simulink model "v1"  (R2025b)
settings: Solver=VariableStepAuto  StartTime=0.0  StopTime=100  RelTol=1e-3
libraries: uavutilslib x1
settings Model: Creator=hamza  LastModifiedBy=hamza

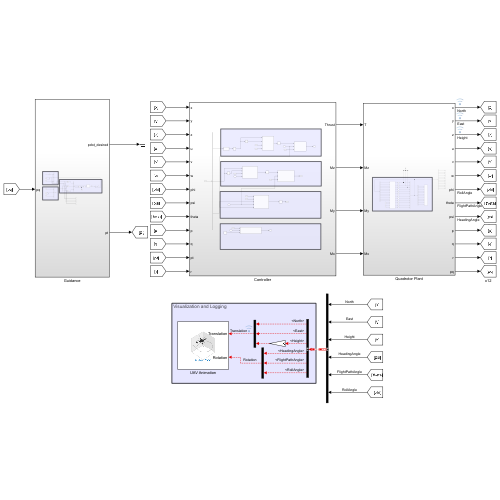
[thumbnail: Simulink's stored preview of the top-level diagram]
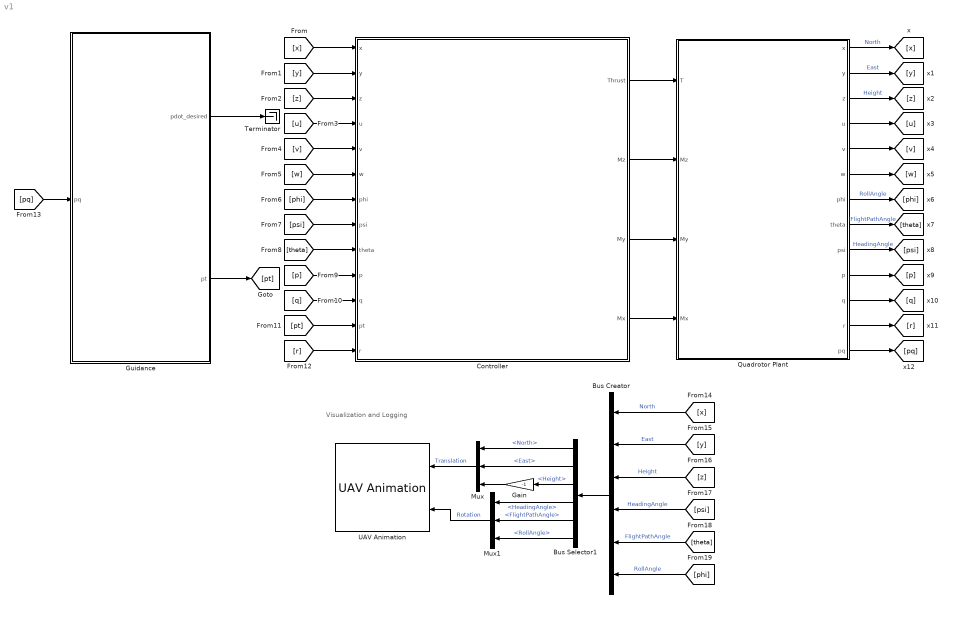
== system v1 ==
  note: Visualization and Logging
  Bus Creator : BusCreator  Inputs=6
  Bus Selector1 : BusSelector  OutputSignals=North,East,Height,HeadingAngle,FlightPathAngle,RollAngle
  Controller : Subsystem
  Gain : Gain  Gain=-1
  Guidance : Subsystem
  Mux : Mux  Inputs=3
  Mux1 : Mux  Inputs=3
  Quadrotor Plant : Subsystem
  Terminator : Terminator
  UAV Animation : uavutilslib/UAV Animation  NumUAV=1  DynamicUAVConfig=off  UAVType=Multirotor  UAVSize=5  UAVColor=[1 0 0]  UAVTrajectoryAlpha=1  InertialZDirection=Down  RotationFormat=Euler ZYX  DrawMarkers=off  SampleTime=0.1
  wires:
  Guidance/1(pdot_desired) -> Terminator/1
  Controller/1(Thrust) -> Quadrotor Plant/1(T)
  Controller/2(Mz) -> Quadrotor Plant/2(Mz)
  Controller/3(My) -> Quadrotor Plant/3(My)
  Controller/4(Mx) -> Quadrotor Plant/4(Mx)
  Mux1/1 -> UAV Animation/2  "Rotation"
  Gain/1 -> Mux/3
  Bus Selector1/1 -> Mux/1  "<North>"
  Bus Selector1/6 -> Mux1/3  "<RollAngle>"
  Mux/1 -> UAV Animation/1  "Translation"
  Bus Selector1/3 -> Gain/1  "<Height>"
  Bus Selector1/2 -> Mux/2  "<East>"
  Bus Selector1/4 -> Mux1/1  "<HeadingAngle>"
  Bus Selector1/5 -> Mux1/2  "<FlightPathAngle>"
  Bus Creator/1 -> Bus Selector1/1
  [x] -> Controller/1(x)
  [y] -> Controller/2(y)
  [z] -> Controller/3(z)
  [u] -> Controller/4(u)
  [v] -> Controller/5(v)
  [w] -> Controller/6(w)
  [phi] -> Controller/7(phi)
  [psi] -> Controller/8(psi)
  [theta] -> Controller/9(theta)
  [p] -> Controller/10(p)
  [q] -> Controller/11(q)
  [pt] -> Controller/12(pt)
  [r] -> Controller/13(r)
  Quadrotor Plant/1(x) -> [x]  "North"
  Quadrotor Plant/2(y) -> [y]  "East"
  Quadrotor Plant/3(z) -> [z]  "Height"
  Quadrotor Plant/4(u) -> [u]
  Quadrotor Plant/5(v) -> [v]
  Quadrotor Plant/6(w) -> [w]
  Quadrotor Plant/7(phi) -> [phi]  "RollAngle"
  Quadrotor Plant/8(theta) -> [theta]  "FlightPathAngle"
  Quadrotor Plant/9(psi) -> [psi]  "HeadingAngle"
  Quadrotor Plant/10(p) -> [p]
  Quadrotor Plant/11(q) -> [q]
  Quadrotor Plant/12(r) -> [r]
  Quadrotor Plant/13(pq) -> [pq]
  Guidance/2(pt) -> [pt]
  [pq] -> Guidance/1(pq)
  [phi] -> Bus Creator/6  "RollAngle"
  [theta] -> Bus Creator/5  "FlightPathAngle"
  [psi] -> Bus Creator/4  "HeadingAngle"
  [z] -> Bus Creator/3  "Height"
  [y] -> Bus Creator/2  "East"
  [x] -> Bus Creator/1  "North"

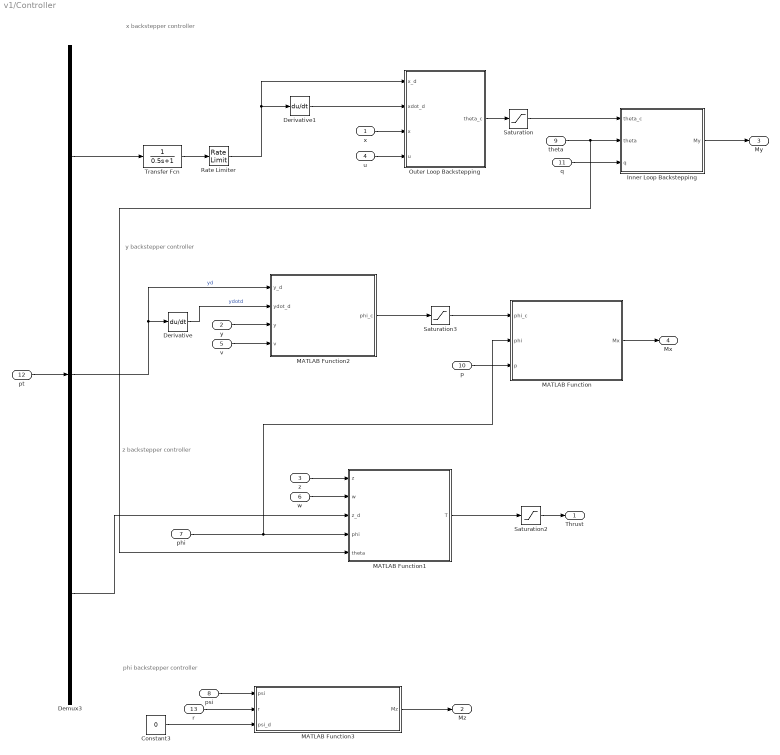
== system v1/Controller ==
  note: phi backstepper controller
  note: z backstepper controller
  note: y backstepper controller
  note: x backstepper controller
  x : Inport
  y : Inport  Port=2
  z : Inport  Port=3
  u : Inport  Port=4
  v : Inport  Port=5
  w : Inport  Port=6
  phi : Inport  Port=7
  psi : Inport  Port=8
  theta : Inport  Port=9
  p : Inport  Port=10
  q : Inport  Port=11
  pt : Inport  Port=12
  r : Inport  Port=13
  Constant3 : Constant  Value=0
  Demux3 : Demux  Outputs=3
  Derivative : Derivative
  Derivative1 : Derivative
  Inner Loop Backstepping : MATLAB Function  TreatAsAtomicUnit=on
  MATLAB Function : MATLAB Function  TreatAsAtomicUnit=on
  MATLAB Function1 : MATLAB Function  TreatAsAtomicUnit=on
  MATLAB Function2 : MATLAB Function  TreatAsAtomicUnit=on
  MATLAB Function3 : MATLAB Function  TreatAsAtomicUnit=on
  Outer Loop Backstepping : MATLAB Function  TreatAsAtomicUnit=on
  Rate Limiter : RateLimiter  RisingSlewLimit=0.5  FallingSlewLimit=-0.5  SampleTimeMode=inherited
  Saturation : Saturate  UpperLimit=0.1  LowerLimit=-0.1
  Saturation2 : Saturate  UpperLimit=22  LowerLimit=0
  Saturation3 : Saturate  UpperLimit=0.1  LowerLimit=-0.1
  Transfer Fcn : TransferFcn  Denominator=[0.5 1]
  Thrust : Outport
  Mz : Outport  Port=2
  My : Outport  Port=3
  Mx : Outport  Port=4
  wires:
  z/1 -> MATLAB Function1/1(z)
  x/1 -> Outer Loop Backstepping/3(x)
  Saturation/1 -> Inner Loop Backstepping/1(theta_c)
  Inner Loop Backstepping/1(My) -> My/1
  Constant3/1 -> MATLAB Function3/3(psi_d)
  Saturation3/1 -> MATLAB Function/1(phi_c)
  phi/1 -> MATLAB Function/2(phi), MATLAB Function1/4(phi)
  Demux3/1 -> Transfer Fcn/1
  Demux3/2 -> MATLAB Function2/1(y_d), Derivative/1  "yd"
  Demux3/3 -> MATLAB Function1/3(z_d)
  MATLAB Function2/1(phi_c) -> Saturation3/1
  r/1 -> MATLAB Function3/2(r)
  MATLAB Function3/1(Mz) -> Mz/1
  y/1 -> MATLAB Function2/3(y)
  Outer Loop Backstepping/1(theta_c) -> Saturation/1
  MATLAB Function1/1(T) -> Saturation2/1
  v/1 -> MATLAB Function2/4(v)
  w/1 -> MATLAB Function1/2(w)
  Derivative/1 -> MATLAB Function2/2(ydot_d)  "ydotd"
  pt/1 -> Demux3/1
  psi/1 -> MATLAB Function3/1(psi)
  u/1 -> Outer Loop Backstepping/4(u)
  theta/1 -> MATLAB Function1/5(theta), Inner Loop Backstepping/2(theta)
  MATLAB Function/1(Mx) -> Mx/1
  q/1 -> Inner Loop Backstepping/3(q)
  p/1 -> MATLAB Function/3(p)
  Saturation2/1 -> Thrust/1
  Derivative1/1 -> Outer Loop Backstepping/2(xdot_d)
  Transfer Fcn/1 -> Rate Limiter/1
  Rate Limiter/1 -> Outer Loop Backstepping/1(x_d), Derivative1/1

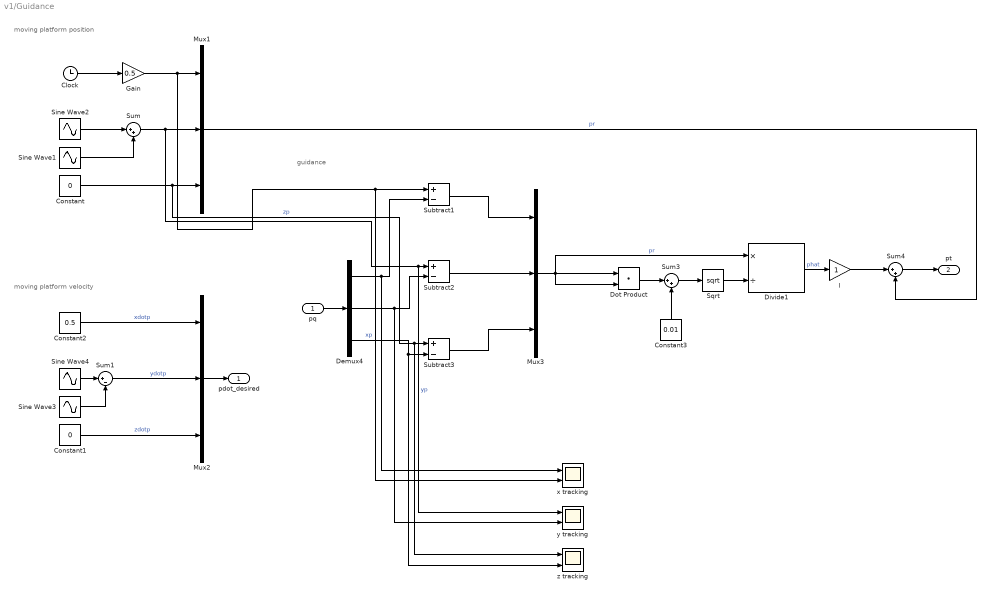
== system v1/Guidance ==
  note: guidance
  note: moving platform position
  note: moving platform velocity
  pq : Inport
  Clock : Clock
  Constant : Constant  Value=0
  Constant1 : Constant  Value=0
  Constant2 : Constant  Value=0.5
  Constant3 : Constant  Value=0.01
  Demux4 : Demux  Outputs=3
  Divide1 : Product  Inputs=*/
  Dot Product : DotProduct  OutDataTypeStr=Inherit: Inherit via internal rule
  Gain : Gain  Gain=0.5
  Mux1 : Mux  Inputs=3
  Mux2 : Mux  Inputs=3
  Mux3 : Mux  Inputs=3
  Sine Wave1 : Sin  Amplitude=2  Frequency=0.2  SampleTime=0
  Sine Wave2 : Sin  Amplitude=2  Frequency=0.2  Phase=pi/2  SampleTime=0
  Sine Wave3 : Sin  Amplitude=0.4  Frequency=0.2  SampleTime=0
  Sine Wave4 : Sin  Amplitude=0.4  Frequency=0.2  Phase=pi/2  SampleTime=0
  Sqrt : Sqrt
  Subtract1 : Sum  Inputs=+-
  Subtract2 : Sum  Inputs=+-
  Subtract3 : Sum  Inputs=+-
  Sum : Sum  Inputs=|++
  Sum1 : Sum  Inputs=|+-
  Sum3 : Sum  Inputs=|++
  Sum4 : Sum  Inputs=|++
  l : Gain
  x tracking : Scope  NumInputPorts=2
      settings: ActiveDisplayYMinimum=-1  ActiveDisplayYMaximum=1  DataLoggingVariableName=ScopeData5
  y tracking : Scope  NumInputPorts=2
      settings: ActiveDisplayYMinimum=-6.2686091559816877  ActiveDisplayYMaximum=6.2529287715888877  DataLoggingVariableName=ScopeData6
  z tracking : Scope  NumInputPorts=2
      settings: ActiveDisplayYMinimum=-1  ActiveDisplayYMaximum=1  DataLoggingVariableName=ScopeData7
  pdot_desired : Outport
  pt : Outport  Port=2
  wires:
  Sine Wave3/1 -> Sum1/2
  Mux1/1 -> Sum4/2  "pr"
  Sine Wave1/1 -> Sum/2
  Constant2/1 -> Mux2/1  "xdotp"
  Constant/1 -> z tracking/1, Subtract3/1, Mux1/3  "zp"
  Sum1/1 -> Mux2/2  "ydotp"
  pq/1 -> Demux4/1
  Sine Wave4/1 -> Sum1/1
  Constant1/1 -> Mux2/3  "zdotp"
  Clock/1 -> Gain/1
  Gain/1 -> x tracking/2, Subtract1/1, Mux1/1  "xp"
  Sum/1 -> y tracking/1, Subtract2/1, Mux1/2  "yp"
  Mux2/1 -> pdot_desired/1
  Sine Wave2/1 -> Sum/1
  Demux4/1 -> x tracking/1, Subtract1/2
  Demux4/2 -> y tracking/2, Subtract2/2
  Demux4/3 -> z tracking/2, Subtract3/2
  Subtract2/1 -> Mux3/2
  Subtract3/1 -> Mux3/3
  Subtract1/1 -> Mux3/1
  Mux3/1 -> Dot Product/1, Divide1/1, Dot Product/2  "pr"
  Dot Product/1 -> Sum3/1
  Constant3/1 -> Sum3/2
  Sum3/1 -> Sqrt/1
  Sqrt/1 -> Divide1/2
  Divide1/1 -> l/1  "phat"
  l/1 -> Sum4/1
  Sum4/1 -> pt/1

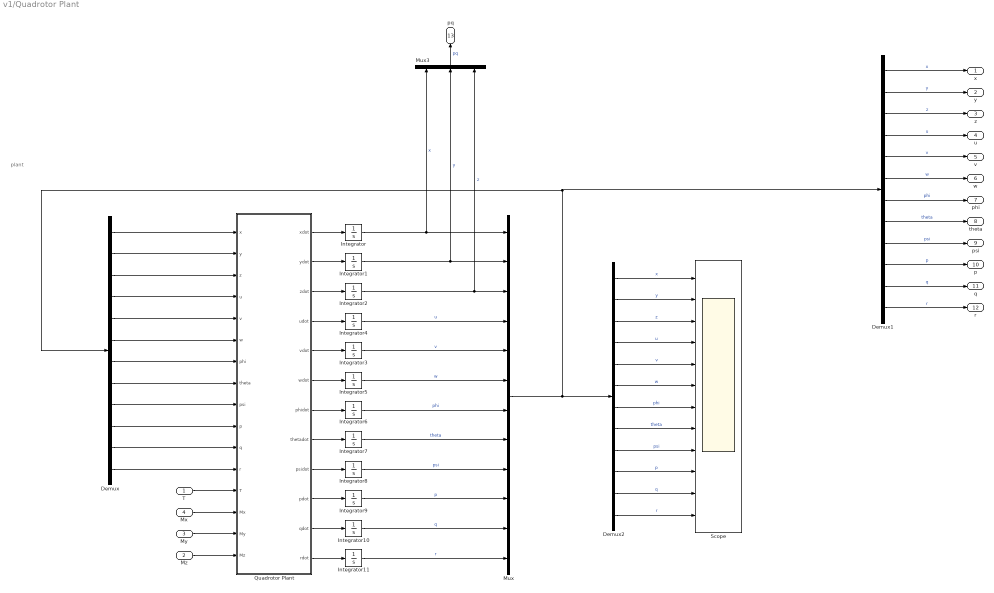
== system v1/Quadrotor Plant ==
  note: plant
  T : Inport
  Mz : Inport  Port=2
  My : Inport  Port=3
  Mx : Inport  Port=4
  Demux : Demux  Outputs=12
  Demux1 : Demux  Outputs=12
  Demux2 : Demux  Outputs=12
  Integrator{,1..11} (12 alike) : Integrator
  Mux : Mux  Inputs=12
  Mux3 : Mux  Inputs=3
  Quadrotor Plant : MATLAB Function  TreatAsAtomicUnit=on
  Scope : Scope  NumInputPorts=12
      settings: ActiveDisplayString=12  ActiveDisplayYMinimum=-1  ActiveDisplayYMaximum=1
  x : Outport
  y : Outport  Port=2
  z : Outport  Port=3
  u : Outport  Port=4
  v : Outport  Port=5
  w : Outport  Port=6
  phi : Outport  Port=7
  theta : Outport  Port=8
  psi : Outport  Port=9
  p : Outport  Port=10
  q : Outport  Port=11
  r : Outport  Port=12
  pq : Outport  Port=13
  wires:
  Demux2/8 -> Scope/8  "theta"
  Demux2/11 -> Scope/11  "q"
  Integrator3/1 -> Mux/5  "v"
  Demux2/5 -> Scope/5  "v"
  Demux/1 -> Quadrotor Plant/1(x)
  Integrator/1 -> Mux/1, Mux3/1  "x"
  Mux/1 -> Demux2/1, Demux1/1, Demux/1
  Integrator2/1 -> Mux3/3, Mux/3  "z"
  Demux/8 -> Quadrotor Plant/8(theta)
  Quadrotor Plant/4(udot) -> Integrator4/1
  Demux/9 -> Quadrotor Plant/9(psi)
  Integrator1/1 -> Mux/2, Mux3/2  "y"
  Demux/6 -> Quadrotor Plant/6(w)
  Quadrotor Plant/12(rdot) -> Integrator11/1
  Quadrotor Plant/5(vdot) -> Integrator3/1
  Demux2/9 -> Scope/9  "psi"
  Integrator5/1 -> Mux/6  "w"
  Quadrotor Plant/9(psidot) -> Integrator8/1
  Demux/4 -> Quadrotor Plant/4(u)
  Demux/12 -> Quadrotor Plant/12(r)
  Quadrotor Plant/2(ydot) -> Integrator1/1
  Mz/1 -> Quadrotor Plant/16(Mz)
  Quadrotor Plant/1(xdot) -> Integrator/1
  Integrator4/1 -> Mux/4  "u"
  Demux2/10 -> Scope/10  "p"
  Demux2/3 -> Scope/3  "z"
  Demux/11 -> Quadrotor Plant/11(q)
  Demux2/6 -> Scope/6  "w"
  Demux/2 -> Quadrotor Plant/2(y)
  Demux2/4 -> Scope/4  "u"
  Integrator8/1 -> Mux/9  "psi"
  Integrator10/1 -> Mux/11  "q"
  Demux/10 -> Quadrotor Plant/10(p)
  Demux2/1 -> Scope/1  "x"
  Quadrotor Plant/10(pdot) -> Integrator9/1
  Mx/1 -> Quadrotor Plant/14(Mx)
  Demux2/2 -> Scope/2  "y"
  Quadrotor Plant/7(phidot) -> Integrator6/1
  Integrator7/1 -> Mux/8  "theta"
  Mux3/1 -> pq/1  "pq"
  Integrator11/1 -> Mux/12  "r"
  Demux2/12 -> Scope/12  "r"
  Demux/5 -> Quadrotor Plant/5(v)
  T/1 -> Quadrotor Plant/13(T)
  Integrator9/1 -> Mux/10  "p"
  Demux/7 -> Quadrotor Plant/7(phi)
  Quadrotor Plant/8(thetadot) -> Integrator7/1
  Quadrotor Plant/3(zdot) -> Integrator2/1
  Demux2/7 -> Scope/7  "phi"
  Demux/3 -> Quadrotor Plant/3(z)
  Quadrotor Plant/6(wdot) -> Integrator5/1
  Quadrotor Plant/11(qdot) -> Integrator10/1
  My/1 -> Quadrotor Plant/15(My)
  Integrator6/1 -> Mux/7  "phi"
  Demux1/1 -> x/1  "x"
  Demux1/2 -> y/1  "y"
  Demux1/3 -> z/1  "z"
  Demux1/4 -> u/1  "u"
  Demux1/5 -> v/1  "v"
  Demux1/6 -> w/1  "w"
  Demux1/7 -> phi/1  "phi"
  Demux1/8 -> theta/1  "theta"
  Demux1/9 -> psi/1  "psi"
  Demux1/10 -> p/1  "p"
  Demux1/11 -> q/1  "q"
  Demux1/12 -> r/1  "r"

== matlab function v1/Controller/MATLAB Function2 ==
  data: y_d input; ydot_d input; phi_c output; y input; v input
function phi_c = y_outer_track(y_d, ydot_d, y, v)

k1y = 0.35;
k2y = 0.55;

phi_c = k1y*(y_d - y) + k2y*(ydot_d - v);

end

== matlab function v1/Controller/MATLAB Function3 ==
  data: psi input; Mz output; r input; psi_d input
function Mz = yaw_backstepping(psi, r, psi_d)

% Gains 
k1 = 1.0;
k2 = 1.5;

% Inertia 
Iz = 7.8187e-5;  

% Step 1: position error
e1 = psi - psi_d;

% Step 2: virtual control 
r_d = -k1 * e1;

% Step 3: velocity error
e2 = r - r_d;

% Step 4: control law
Mz = Iz * ( -k2 * e2 - k1 * r );

end

== matlab function v1/Controller/Inner Loop Backstepping ==
  data: theta_c input; My output; theta input; q input
function My = inner_pitch_pd(theta_c, theta, q)

Kp = 10;
Kd = 6;

My_unsat = Kp * (theta_c - theta) - Kd * q;

My_lim = 0.25;

if My_unsat > My_lim
    My = My_lim;
elseif My_unsat < -My_lim
    My = -My_lim;
else
    My = My_unsat;
end

end

== matlab function v1/Quadrotor Plant/Quadrotor Plant ==
  data: x input; y input; z input; u input; xdot output; v input; w input; phi input; theta input; psi input; p input; q input; r input; T input; Mx input; My input; Mz input; ydot output; zdot output; udot output; vdot output; wdot output; phidot output; thetadot output; psidot output; pdot output; qdot output; rdot output
function [xdot,ydot,zdot,udot,vdot,wdot,phidot,thetadot,psidot,pdot,qdot,rdot] = quadPlant(x,y,z,u,v,w,phi,theta,psi,p,q,r,T,Mx,My,Mz)

% Parameters
m = 1.1;
g = 9.8;

Ix = 0.013;
Iy = 0.024;
Iz = 7.8187e-5;

% Disturbances (start with zero)
fdx = 0;
fdy = 0;
fdz = 0;

tdx = 0;
tdy = 0;
tdz = 0;

% Rotation matrix: body to inertial
cphi = cos(phi);   sphi = sin(phi);
cth  = cos(theta); sth  = sin(theta);
cpsi = cos(psi);   spsi = sin(psi);

R = [ cth*cpsi,  sphi*sth*cpsi - cphi*spsi,  cphi*sth*cpsi + sphi*spsi;
      cth*spsi,  sphi*sth*spsi + cphi*cpsi,  cphi*sth*spsi - sphi*cpsi;
      -sth,      sphi*cth,                   cphi*cth                 ];

% Angular velocity skew-symmetric matrix
S = [  0  -r   q;
       r   0  -p;
      -q   p   0 ];

% Body linear velocity vector
vB = [u; v; w];

% Position derivatives in inertial frame
pIdot = R * vB;
xdot = pIdot(1);
ydot = pIdot(2);
zdot = pIdot(3);

% External force in body frame
% fext = -T*e3 + m*g*(R')*e3 + fd
e3 = [0;0;1];
fd = [fdx; fdy; fdz];
fext = -T*e3 + m*g*(R')*e3 + fd;

% Linear acceleration in body frame
vBdot = -S*vB + (1/m)*fext;
udot = vBdot(1);
vdot = vBdot(2);
wdot = vBdot(3);

% Euler angle rate matrix
% [phi_dot; theta_dot; psi_dot] = Psi * [p;q;r]
% Avoid theta near +-pi/2
eps_val = 1e-6;
if abs(cth) < eps_val
    cth = eps_val * sign(cth + eps_val);
end

Psi = [1, sphi*tan(theta), cphi*tan(theta);
       0, cphi,           -sphi;
       0, sphi/cth,        cphi/cth];

etaDot = Psi * [p; q; r];
phidot   = etaDot(1);
thetadot = etaDot(2);
psidot   = etaDot(3);

% Angular dynamics
J = diag([Ix Iy Iz]);
wB = [p; q; r];
M  = [Mx; My; Mz];
td = [tdx; tdy; tdz];

wBdot = J \ (-S*(J*wB) + M + td);

pdot = wBdot(1);
qdot = wBdot(2);
rdot = wBdot(3);
end

== matlab function v1/Controller/Outer Loop Backstepping ==
  data: x_d input; xdot_d input; x input; theta_c output; u input
function theta_c = x_outer(x_d, xdot_d, x, u)

k1x = 0.04;
k2x = 0.12;

theta_c = -k1x*(x_d - x) - k2x*(xdot_d - u);
end

== matlab function v1/Controller/MATLAB Function1 ==
  data: z input; T output; w input; z_d input; phi input; theta input
function T = z_backstepping(z, w, z_d, phi, theta)

% Gains
k1 = 1.0;
k2 = 1.5;

% Parameters
m = 1.1;
g = 9.8;

% Safety for tilt compensation
eps_val = 0.01;
c = cos(phi)*cos(theta);

if abs(c) < eps_val
    c = eps_val * sign(c + eps_val);
end

% Errors
e1 = z - z_d;
w_d = -k1 * e1;
e2 = w - w_d;

% Correct thrust law for this plant
T = (m / c) * ( g + k2*e2 + k1*w );

end

== matlab function v1/Controller/MATLAB Function ==
  data: phi_c input; phi input; p input; Mx output
function Mx = roll_pd(phi_c, phi, p)

kp = 6;
kd = 3.5;

Mx = kp*(phi_c - phi) - kd*p;

end
